simulink model "Visual6dof"  (R2017b)
settings: Solver=FixedStepDiscrete  StartTime=0.0  StopTime=100000  FixedStep=.1  RelTol=1e-3  EnableMultiTasking=on
undefined symbols (not defined in the file or in its folder): Visualisation
libraries: simulink x6
settings Model: Creator=b6034940  LastModifiedBy=fahim
settings DataIOCC: LimitDataPoints=on  SaveFormat=Array
settings OptimizationCC: InitFltsAndDblsToZero=on  LifeSpan=inf
settings CodeAppCC: StateflowObjectComments=on

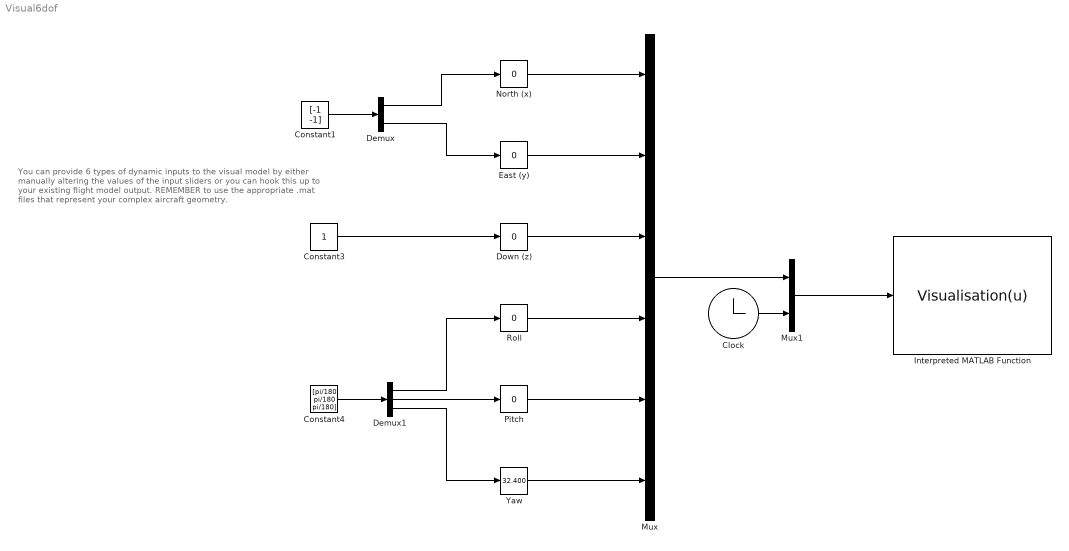
== system Visual6dof ==
  note: You can provide 6 types of dynamic inputs
      | to the visual model by either manually
      | altering the values of the input sliders
      | or you can hook this up to your existing
      | flight model output.
      |
      | REMEMBER to use the appropriate .mat files that represent your complex aircraft geometry.
  Clock : Clock
  Constant1 : Constant  Value=[-1 -1]
  Constant3 : Constant
  Constant4 : Constant  Value=[pi/180 pi/180 pi/180]
  Demux : Demux  Outputs=2
  Demux1 : Demux  Outputs=3
  Down (z) : simulink/Math Operations/Slider Gain  gain=0  low=-100  high=100
  East (y) : simulink/Math Operations/Slider Gain  gain=0  low=-100  high=100
  Interpreted MATLAB Function : MATLABFcn  MATLABFcn=Visualisation(u)  OutputDimensions=0
  Mux : Mux  Inputs=6
  Mux1 : Mux  Inputs=2
  North (x) : simulink/Math Operations/Slider Gain  gain=0  low=-100  high=100
  Pitch : simulink/Math Operations/Slider Gain  gain=0  low=-180  high=180
  Roll : simulink/Math Operations/Slider Gain  gain=0  low=-180  high=180
  Yaw : simulink/Math Operations/Slider Gain  gain=32.400  low=-180  high=180
  wires:
  Constant1/1 -> Demux/1
  Constant3/1 -> Down (z)/1
  North (x)/1 -> Mux/1
  East (y)/1 -> Mux/2
  Down (z)/1 -> Mux/3
  Roll/1 -> Mux/4
  Pitch/1 -> Mux/5
  Yaw/1 -> Mux/6
  Mux/1 -> Mux1/1
  Clock/1 -> Mux1/2
  Mux1/1 -> Interpreted MATLAB Function/1
  Demux/1 -> North (x)/1
  Demux/2 -> East (y)/1
  Constant4/1 -> Demux1/1
  Demux1/2 -> Pitch/1
  Demux1/1 -> Roll/1
  Demux1/3 -> Yaw/1
